simulink model "ards_model"  (R2020b)
settings: Solver=VariableStepAuto  StartTime=0.0  StopTime=480  MaxStep=0.2  RelTol=1e-3
model workspace: external: MAT-File model_workspace.mat (data not in the file)
values from neighbouring files (symbols this model uses):
  C_a_CO2_0 = 0.54    [model_workspace.mat]
  C_a_O2_0 = 0.1974    [model_workspace.mat]
  C_v_CO2_0 = 0.72    [model_workspace.mat]
  C_v_O2_0 = 0.13    [model_workspace.mat]
  moving_average_period = 5    [model_workspace.mat]
  P_ap_0 = 15    [model_workspace.mat]
  P_as_0 = 105.55    [model_workspace.mat]
  P_default = [105.55 4 15 6]    [model_workspace.mat]
  P_vs_0 = 4    [model_workspace.mat]
  Q_0 = 4.8    [model_workspace.mat]
undefined symbols (not defined in the file or in its folder): cRS, Pinsp, VT
libraries: pid_lib x1
(part 3 of 3)

== system ards_model/main-model/Lung volume model/Inspiratory lung volume derivative (fourier approximation)/Half-wave rectifier ==
  (d)VA : Inport
  2pift : Inport  Port=2
  Add : Sum  Inputs=+-+
  Add2 : Sum  Inputs=+++
  Constant : Constant  Value=1/pi
  Constant1 : Constant  Value=2
  Constant2 : Constant  Value=4
  Constant3 : Constant  Value=6
  Gain : Gain  Gain=1/2
  Gain1 : Gain  Gain=2/pi
  Product1 : Product
  Trigonometric Function : Trigonometry
  summand (k=2) : Subsystem
  summand (k=4) : Subsystem
  summand (k=6) : Subsystem
  out : Outport
  wires:
  Trigonometric Function/1 -> Gain/1
  Gain/1 -> Add/3
  (d)VA/1 -> Product1/2  "A"
  2pift/1 -> summand (k=6)/1(In1), summand (k=4)/1(In1), summand (k=2)/1(In1), Trigonometric Function/1  "omega*t"
  Constant/1 -> Add/1
  Add/1 -> Product1/1
  Product1/1 -> out/1
  Gain1/1 -> Add/2
  Add2/1 -> Gain1/1
  Constant1/1 -> summand (k=2)/2(In2)
  summand (k=2)/1(Out1) -> Add2/1
  summand (k=4)/1(Out1) -> Add2/2
  summand (k=6)/1(Out1) -> Add2/3
  Constant3/1 -> summand (k=6)/2(In2)
  Constant2/1 -> summand (k=4)/2(In2)

== system ards_model/main-model/Predicted Body Weight/IfThenElse/Subsystem1 ==
  in : Inport
  Enable : EnablePort
  out : Outport
  wires:
  in/1 -> out/1

== system ards_model/main-model/Predicted Body Weight/IfThenElse/Subsystem2 ==
  in : Inport
  Enable : EnablePort
  out : Outport
  wires:
  in/1 -> out/1

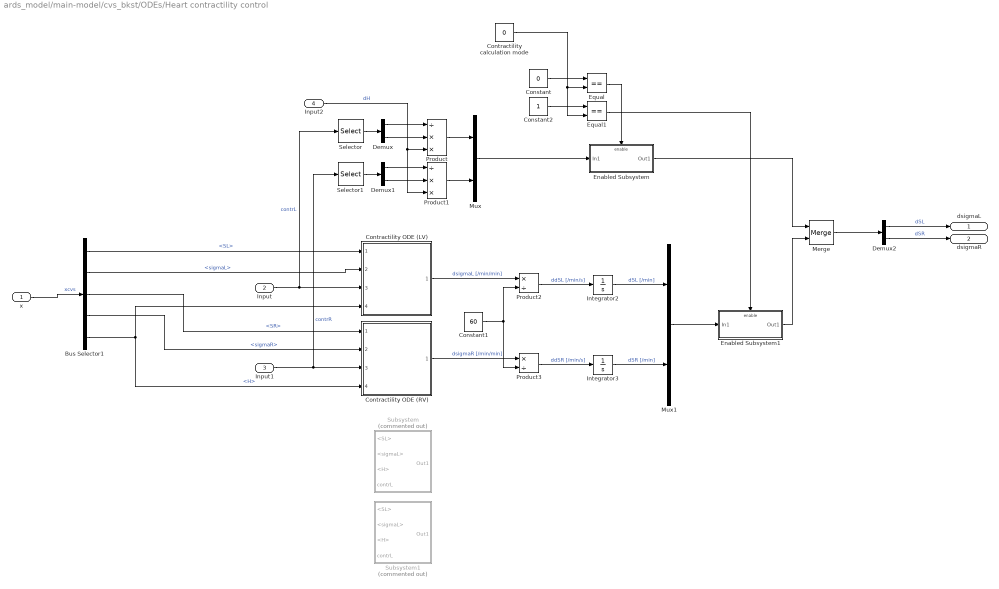
== system ards_model/main-model/cvs_bkst/ODEs/Heart contractility control ==
  x : Inport  OutDataTypeStr=Bus: CardioVascularState
  Input : Inport  Port=2  OutDataTypeStr=double  PortDimensions=3
  Input1 : Inport  Port=3  OutDataTypeStr=double  PortDimensions=3
  Input2 : Inport  Port=4  Unit=1/min^2
  Bus Selector1 : BusSelector  OutputSignals=SL,sigmaL,SR,sigmaR,H
  Constant : Constant  Value=0
  Constant1 : Constant  Value=60
  Constant2 : Constant
  Contractility ODE (LV) : Subsystem  ReferencedSubsystem=cvrs_contractility_control
  Contractility ODE (RV) : Subsystem  ReferencedSubsystem=cvrs_contractility_control
  Contractility calculation mode : Constant  Value=0
  Demux : Demux  Outputs=2
  Demux1 : Demux  Outputs=2
  Demux2 : Demux  Outputs=2
  Enabled Subsystem : Subsystem  TreatAsAtomicUnit=on
  Enabled Subsystem1 : Subsystem  TreatAsAtomicUnit=on
  Equal : RelationalOperator  Operator===  OutDataTypeStr=boolean  RndMeth=Simplest
  Equal1 : RelationalOperator  Operator===  OutDataTypeStr=boolean  RndMeth=Simplest
  Integrator2 : Integrator
  Integrator3 : Integrator
  Merge : Merge
  Mux : Mux  Inputs=2
  Mux1 : Mux  Inputs=2
  Product : Product  Inputs=/**
  Product1 : Product  Inputs=/**
  Product2 : Product  Inputs=*/
  Product3 : Product  Inputs=*/
  Selector : Selector  InputPortWidth=3  IndexOptions=Index vector (dialog)  Indices=[1 2]  OutputSizes=1
  Selector1 : Selector  InputPortWidth=3  IndexOptions=Index vector (dialog)  Indices=[1 2]  OutputSizes=1
  Subsystem : Subsystem  Commented=on
  Subsystem1 : Subsystem  Commented=on
  dsigmaL : Outport  Unit=mmHg/min
  dsigmaR : Outport  Port=2  Unit=mmHg/min
  wires:
  Integrator3/1 -> Mux1/2  "dSR [/min]"
  Integrator2/1 -> Mux1/1  "dSL [/min]"
  Product3/1 -> Integrator3/1  "ddSR [/min/s]"
  Product2/1 -> Integrator2/1  "ddSL [/min/s]"
  Constant1/1 -> Product2/2, Product3/2
  Bus Selector1/3 -> Contractility ODE (RV)/1  "<SR>"
  Input1/1 -> Selector1/1, Contractility ODE (RV)/3  "contrR"
  Contractility ODE (LV)/1 -> Product2/1  "dsigmaL [/min/min]"
  Input/1 -> Selector/1, Contractility ODE (LV)/3  "contrL"
  Bus Selector1/1 -> Contractility ODE (LV)/1  "<SL>"
  Contractility ODE (RV)/1 -> Product3/1  "dsigmaR [/min/min]"
  x/1 -> Bus Selector1/1  "xcvs"
  Bus Selector1/4 -> Contractility ODE (RV)/2  "<sigmaR>"
  Bus Selector1/2 -> Contractility ODE (LV)/2  "<sigmaL>"
  Bus Selector1/5 -> Contractility ODE (LV)/4, Contractility ODE (RV)/4  "<H>"
  Selector/1 -> Demux/1
  Demux/1 -> Product/1
  Demux/2 -> Product/2
  Demux1/2 -> Product1/2
  Demux1/1 -> Product1/1
  Selector1/1 -> Demux1/1
  Product/1 -> Mux/1
  Product1/1 -> Mux/2
  Mux/1 -> Enabled Subsystem/1(In1)
  Mux1/1 -> Enabled Subsystem1/1(In1)
  Equal/1 -> Enabled Subsystem/Enable
  Equal1/1 -> Enabled Subsystem1/Enable
  Enabled Subsystem/1(Out1) -> Merge/1
  Enabled Subsystem1/1(Out1) -> Merge/2
  Demux2/1 -> dsigmaL/1  "dSL"
  Demux2/2 -> dsigmaR/1  "dSR"
  Merge/1 -> Demux2/1
  Constant/1 -> Equal/1
  Constant2/1 -> Equal1/1
  Contractility calculation mode/1 -> Equal1/2, Equal/2
  Input2/1 -> Product1/3, Product/3  "dH"

== system ards_model/main-model/cvs_bkst/ODEs/Heart rate control ==
  <Pas> : Inport  Unit=mmHg
  ABP error term : Subsystem
  Lung-to-carotid delay [BKST] ch. 2.3.1 : TransportDelay  DelayTime=6
  PID Controller : pid_lib/PID Controller  Controller=PID  Form=Parallel  TimeDomain=Continuous-time  UseExternalTs=off  SampleTime=-1  IntegratorMethod=Forward Euler  FilterMethod=Forward Euler  ControllerParametersSource=internal  P=0.5  I=0  D=-0.3  UseFilter=on  N=100  TunerSelectOption=Transfer Function Based (PID Tuner App)  InitialConditionSource=internal  InitialConditionForIntegrator=0  InitialConditionForFilter=0  DifferentiatorICPrevScaledInput=0  ExternalReset=none  TrackingMode=off  Kt=1  LimitOutput=off  SatLimitsSource=internal  UpperSaturationLimit=inf  LowerSaturationLimit=-inf  LinearizeAsGain=on  AntiWindupMode=none  Kb=1  POutMin=[]  POutMax=[]  IOutMin=[]  IOutMax=[]  DOutMin=[]  DOutMax=[]  NOutMin=[]  NOutMax=[]  SumOutMin=[]  SumOutMax=[]  SaturationOutMin=[]  SaturationOutMax=[]  PParamMin=[]  PParamMax=[]  IParamMin=[]  IParamMax=[]  DParamMin=[]  DParamMax=[]  NParamMin=[]  NParamMax=[]  KbParamMin=[]  KbParamMax=[]  KtParamMin=[]  KtParamMax=[]  KbOutMin=[]  KbOutMax=[]  KtOutMin=[]  KtOutMax=[]  IntegratorOutMin=[]  IntegratorOutMax=[]  FilterOutMin=[]  FilterOutMax=[]  SumI1OutMin=[]  SumI1OutMax=[]  SumI2OutMin=[]  SumI2OutMax=[]  SumI3OutMin=[]  SumI3OutMax=[]  SumI4OutMin=[]  SumI4OutMax=[]  SumDOutMin=[]  SumDOutMax=[]  DifferentiatorOutMin=[]  DifferentiatorOutMax=[]  FilterDiffOutCoefMin=[]  FilterDiffOutCoefMax=[]  ReciprocalOutMin=[]  ReciprocalOutMax=[]  SumDenOutMin=[]  SumDenOutMax=[]  SumNumOutMin=[]  SumNumOutMax=[]  DivideOutMin=[]  DivideOutMax=[]  UdiffTsProdOutMin=[]  UdiffTsProdOutMax=[]  NTsProdOutMin=[]  NTsProdOutMax=[]  UintegralTsProdOutMin=[]  UintegralTsProdOutMax=[]  UngainTsProdOutMin=[]  UngainTsProdOutMax=[]  IntegratorContinuousStateAttributes=''  IntegratorStateMustResolveToSignalObject=off  IntegratorRTWStateStorageClass=Auto  FilterContinuousStateAttributes=''  FilterStateMustResolveToSignalObject=off  FilterRTWStateStorageClass=Auto  ParallelPVariant=InternalParameters  IdealPVariant=Disabled  IVariant=InternalParameters  DVariant=InternalParameters  IntegratorVariant=Continuous  SatVariant=Disabled  AWVariant=Passthrough  PCopyVariant=Disabled  TRVariant=Disabled  FdbkBlocksVariant=Forward  IdealPFdbkVariant=Disabled  SatFdbkVariant=Disabled  DerivativeFilterVariant=ContFilter  NVariant=InternalParameters  NCopyVariant=Disabled  FilterICVariant=InternalICsFilter  IntegratorICVariant=InternalICs  ExternalResetVariant=Disabled  TRSumVariant=Passthrough  SumFdbkVariant=Disabled  SumVariant=Sum_PID  TsampFilterVariant=InternalTs  TsampNgainVariant=Passthrough  TsampIntegralVariant=Passthrough  ExternalSaturationOutDataTypeStr=Inherit: Same as second input
  Pas : Constant  Value=105.5
  dH [/min] : Outport  Unit=1/min^2
  wires:
  ABP error term/1(Out1) -> Lung-to-carotid delay [BKST] ch. 2.3.1/1
  PID Controller/1 -> dH [/min]/1  "dH [/min]"
  <Pas>/1 -> ABP error term/1(<Pas>)  "Pas"
  Pas/1 -> ABP error term/2(<Pas>1)
  Lung-to-carotid delay [BKST] ch. 2.3.1/1 -> PID Controller/1

== system ards_model/main-model/cvs_bkst/ODEs/Systemic vascular resistance control ==
  xcvsExt : Inport  OutDataTypeStr=Bus: CardioVascularStateExtended
  Ca;O2 : Inport  Port=2  Unit=1
  Ca;O1 : Inport  Port=3  Unit=1
  -MR_;O2 : Inport  Port=4  Unit=L/min
  Apesk [mmHg*min/L] : Constant  Value=178
  Bus Selector : BusSelector  OutputSignals=Qs,Pas,Pvs
  Constant3 : Constant  Value=0
  Derivative : Derivative
  Divide1 : Product  Inputs=*/
  K [L] : Constant  Value=15.9591
  Product : Product
  Product1 : Product
  Product2 : Product
  Subsystem : Subsystem
  Subtract : Sum  Inputs=+-
  Subtract1 : Sum  Inputs=+-
  Subtract2 : Sum  Inputs=+-
  Rs1 : Outport  Unit=mmHg/L
  wires:
  -MR_;O2/1 -> Subtract1/2  "-MR_;O2"
  Product1/1 -> Subtract2/1
  Product/1 -> Subtract1/1
  Subtract2/1 -> Divide1/1
  Subtract1/1 -> Product1/2
  Subtract/1 -> Subtract2/2  "deltaP"
  Ca;O2/1 -> Product/1  "Ca;O2"
  Bus Selector/2 -> Subtract/1  "<Pas>"
  Bus Selector/1 -> Product/2  "<Qs>"
  Apesk [mmHg*min/L]/1 -> Product1/1, Product2/1  "Apesk"
  K [L]/1 -> Divide1/2  "K"
  xcvsExt/1 -> Bus Selector/1  "xcvsExt"
  Bus Selector/3 -> Subtract/2  "<Pvs>"
  Ca;O1/1 -> Derivative/1  "Cv;O2"
  Derivative/1 -> Product2/2
  Constant3/1 -> Subsystem/1(dRs [0])
  Product2/1 -> Subsystem/2(dRs [v])  "dRs [v]"
  Divide1/1 -> Subsystem/3(dRs [a])  "dRs [a]"
  Subsystem/1(dRs) -> Rs1/1  "dRs"

== system ards_model/main-model/cvs_bkst/ODEs/Vessel pressure control (ap) ==
  Qin : Inport
  Qout : Inport  Port=2
  c_ : Inport  Port=3
  Add4 : Sum  Inputs=+-
  Product4 : Product  Inputs=*/
  dP_ : Outport
  wires:
  Qout/1 -> Add4/2
  Product4/1 -> dP_/1  "dP_"
  c_/1 -> Product4/2
  Qin/1 -> Add4/1
  Add4/1 -> Product4/1

== system ards_model/main-model/cvs_bkst/ODEs/Vessel pressure control (as) ==
  Qin : Inport
  Qout : Inport  Port=2
  c_ : Inport  Port=3
  Add4 : Sum  Inputs=+-
  Product4 : Product  Inputs=*/
  dP_ : Outport
  wires:
  Add4/1 -> Product4/1
  Qin/1 -> Add4/1
  c_/1 -> Product4/2
  Product4/1 -> dP_/1  "dP_"
  Qout/1 -> Add4/2

== system ards_model/main-model/cvs_bkst/ODEs/Vessel pressure control (vs) ==
  Qin : Inport
  Qout : Inport  Port=2
  c_ : Inport  Port=3
  Add4 : Sum  Inputs=+-
  Product4 : Product  Inputs=*/
  dP_ : Outport
  wires:
  Add4/1 -> Product4/1
  Qin/1 -> Add4/1
  c_/1 -> Product4/2
  Product4/1 -> dP_/1  "dP_"
  Qout/1 -> Add4/2

== system ards_model/main-model/rs_tehrani/ODEs/Ambient air pressure (-H2O) ==
  QT12 : Inport
  PA;H2O [mmHg] : Constant  Value=47
  Subtract : Sum  Inputs=+-
  Output : Outport
  wires:
  QT12/1 -> Subtract/1  "Pamb"
  PA;H2O [mmHg]/1 -> Subtract/2
  Subtract/1 -> Output/1  "Pamb*"

== system ards_model/main-model/rs_tehrani/ODEs/Insipired gas pressures ==
  Pamb* : Inport  Unit=mmHg
  Fi;O2 : Inport  Port=2  Unit=1
  Fi;CO2 : Inport  Port=3  Unit=1
  Product : Product  Inputs=**
  Product1 : Product  Inputs=**
  Pi;O2 : Outport  Unit=mmHg
  Pi;CO2 : Outport  Port=2  Unit=mmHg
  wires:
  Fi;CO2/1 -> Product1/2
  Fi;O2/1 -> Product/2
  Product/1 -> Pi;O2/1  "Pi;O2"
  Product1/1 -> Pi;CO2/1  "Pi;CO2"
  Pamb*/1 -> Product/1, Product1/1

== system ards_model/main-model/rs_tehrani/ODEs/lung_compartment ==
  Pamb* : Inport  Unit=mmHg
  dv1 : Inport  Port=2  Unit=L
  dv : Inport  Port=3  Unit=L/s
  Pi;O2 : Inport  Port=4  Unit=mmHg
  Pi;CO2 : Inport  Port=5  Unit=mmHg
  Input : Inport  Port=6  OutDataTypeStr=Bus: RespiratoryStateExtended
  dv4 : Inport  Port=7  OutDataTypeStr=Bus: BloodGasFlow
  Bus Selector : BusSelector  OutputSignals=CaxO2,PaxO2
  Bus Selector1 : BusSelector  OutputSignals=CaxCO2,PaxCO2
  Bus Selector2 : BusSelector  OutputSignals=Q,C_O2
  Bus Selector3 : BusSelector  OutputSignals=Q,C_CO2
  CO2 : Subsystem  ReferencedSubsystem=tehrani_alv_mass_balance_v5
  Input1 : InportShadow  Port=6  OutDataTypeStr=Bus: RespiratoryStateExtended
  O2 : Subsystem  ReferencedSubsystem=tehrani_alv_mass_balance_v5
  PA-a;CO2 : Constant  Value=0
  PA-a;O2 : Constant  Value=4
  dv2 : InportShadow  Port=7  OutDataTypeStr=Bus: BloodGasFlow
  Output : Outport  Unit=mmHg/s
  Output1 : Outport  Port=2  Unit=mmHg/s
  wires:
  Bus Selector2/1 -> O2/1  "<Q>"
  Bus Selector2/2 -> O2/2  "<C_O2>"
  Pi;CO2/1 -> CO2/6  "Pi;CO2"
  Bus Selector1/1 -> CO2/3  "<CaxCO2>"
  dv4/1 -> Bus Selector2/1  "inpp*"
  Input1/1 -> Bus Selector1/1  "xrsExt"
  dv2/1 -> Bus Selector3/1  "inpp*"
  Bus Selector3/1 -> CO2/1  "<Q>"
  Bus Selector3/2 -> CO2/2  "<C_CO2>"
  Input/1 -> Bus Selector/1  "xrsExt"
  Bus Selector1/2 -> CO2/4  "<PaxCO2>"
  O2/1 -> Output/1  "dPax;O2"
  Bus Selector/1 -> O2/3  "<CaxO2>"
  PA-a;CO2/1 -> CO2/9  "PA-a;CO2"
  CO2/1 -> Output1/1  "dPax;CO2"
  Bus Selector/2 -> O2/4  "<PaxO2>"
  dv1/1 -> CO2/7, O2/7  "v"
  Pi;O2/1 -> O2/6  "Pi;O2"
  dv/1 -> CO2/8, O2/8  "dv+"
  Pamb*/1 -> CO2/5, O2/5  "Pamb*"
  PA-a;O2/1 -> O2/9  "PA-a;O2"

== system ards_model/ards_classification/Berlin definition/ards_level/ards_level_string/Subsystem ==
  in : Inport
  Enable : EnablePort
  out : Outport
  wires:
  in/1 -> out/1

== system ards_model/ards_classification/Berlin definition/ards_level/ards_level_string/Subsystem1 ==
  in : Inport
  Enable : EnablePort
  out : Outport
  wires:
  in/1 -> out/1

== system ards_model/ards_classification/Berlin definition/ards_level/ards_level_string/Subsystem2 ==
  in : Inport
  Enable : EnablePort
  out : Outport
  wires:
  in/1 -> out/1

== system ards_model/ards_classification/Berlin definition/ards_level/ards_level_string/Subsystem3 ==
  in : Inport
  Enable : EnablePort
  out : Outport
  wires:
  in/1 -> out/1

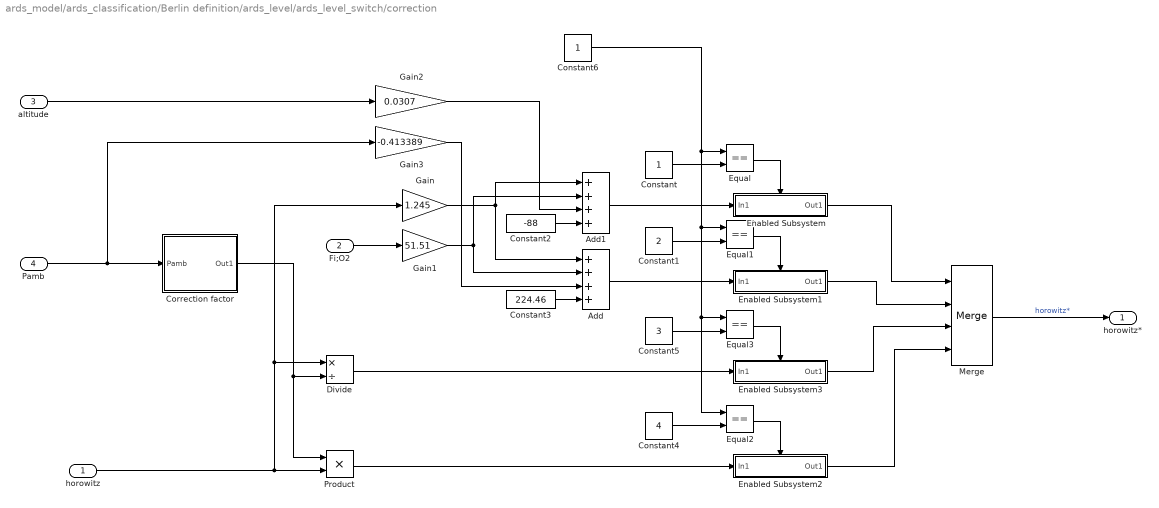
== system ards_model/ards_classification/Berlin definition/ards_level/ards_level_switch/correction ==
  horowitz : Inport
  Fi;O2 : Inport  Port=2
  altitude : Inport  Port=3
  Pamb : Inport  Port=4
  Add : Sum  Inputs=++++
  Add1 : Sum  Inputs=++++
  Constant : Constant
  Constant1 : Constant  Value=2
  Constant2 : Constant  Value=-88
  Constant3 : Constant  Value=224.46
  Constant4 : Constant  Value=4
  Constant5 : Constant  Value=3
  Constant6 : Constant
  Correction factor : Subsystem
  Divide : Product  Inputs=*/
  Enabled Subsystem : Subsystem  TreatAsAtomicUnit=on
  Enabled Subsystem1 : Subsystem  TreatAsAtomicUnit=on
  Enabled Subsystem2 : Subsystem  TreatAsAtomicUnit=on
  Enabled Subsystem3 : Subsystem  TreatAsAtomicUnit=on
  Equal{,1..3} (4 alike) : RelationalOperator  Operator===  OutDataTypeStr=boolean  RndMeth=Simplest
  Gain : Gain  Gain=1.245
  Gain1 : Gain  Gain=51.51
  Gain2 : Gain  Gain=0.0307
  Gain3 : Gain  Gain=-0.413389
  Merge : Merge  Inputs=4
  Product : Product
  horowitz* : Outport
  wires:
  Correction factor/1(Out1) -> Divide/2, Product/1
  Constant1/1 -> Equal1/2
  Constant/1 -> Equal/2
  Constant6/1 -> Equal2/1, Equal3/1, Equal1/1, Equal/1
  Gain1/1 -> Add1/2, Add/2
  horowitz/1 -> Gain/1, Divide/1, Product/2
  Enabled Subsystem/1(Out1) -> Merge/1
  Gain3/1 -> Add/3
  Constant4/1 -> Equal2/2
  Pamb/1 -> Gain3/1, Correction factor/1(Pamb)
  Enabled Subsystem2/1(Out1) -> Merge/4
  Constant2/1 -> Add1/4
  Merge/1 -> horowitz*/1  "horowitz*"
  altitude/1 -> Gain2/1
  Gain/1 -> Add/1, Add1/1
  Add/1 -> Enabled Subsystem1/1(In1)
  Divide/1 -> Enabled Subsystem3/1(In1)
  Enabled Subsystem3/1(Out1) -> Merge/3
  Constant3/1 -> Add/4
  Equal1/1 -> Enabled Subsystem1/Enable
  Add1/1 -> Enabled Subsystem/1(In1)
  Gain2/1 -> Add1/3
  Product/1 -> Enabled Subsystem2/1(In1)
  Equal2/1 -> Enabled Subsystem2/Enable
  Equal3/1 -> Enabled Subsystem3/Enable
  Equal/1 -> Enabled Subsystem/Enable
  Constant5/1 -> Equal3/2
  Enabled Subsystem1/1(Out1) -> Merge/2
  Fi;O2/1 -> Gain1/1

== system ards_model/main-model/Lung volume model/Inspiratory lung volume derivative (fourier approximation)/Half-wave rectifier/summand (k=2) ==
  In1 : Inport
  In2 : Inport  Port=2
  Add1 : Sum  Inputs=+-
  Constant2 : Constant
  Product : Product
  Product3 : Product  Inputs=*/
  Square : Math  Operator=square  SaturateOnIntegerOverflow=on
  Trigonometric Function1 : Trigonometry  Operator=cos
  Out1 : Outport
  wires:
  Add1/1 -> Product3/2
  Trigonometric Function1/1 -> Product3/1
  Square/1 -> Add1/1
  In1/1 -> Product/1  "omega*t"
  In2/1 -> Product/2, Square/1  "n"
  Product/1 -> Trigonometric Function1/1
  Product3/1 -> Out1/1
  Constant2/1 -> Add1/2

== system ards_model/main-model/Lung volume model/Inspiratory lung volume derivative (fourier approximation)/Half-wave rectifier/summand (k=4) ==
  In1 : Inport
  In2 : Inport  Port=2
  Add1 : Sum  Inputs=+-
  Constant2 : Constant
  Product : Product
  Product3 : Product  Inputs=*/
  Square : Math  Operator=square  SaturateOnIntegerOverflow=on
  Trigonometric Function1 : Trigonometry  Operator=cos
  Out1 : Outport
  wires:
  Constant2/1 -> Add1/2
  Product3/1 -> Out1/1
  Product/1 -> Trigonometric Function1/1
  In2/1 -> Square/1, Product/2  "n"
  In1/1 -> Product/1  "omega*t"
  Square/1 -> Add1/1
  Trigonometric Function1/1 -> Product3/1
  Add1/1 -> Product3/2

== system ards_model/main-model/Lung volume model/Inspiratory lung volume derivative (fourier approximation)/Half-wave rectifier/summand (k=6) ==
  In1 : Inport
  In2 : Inport  Port=2
  Add1 : Sum  Inputs=+-
  Constant2 : Constant
  Product : Product
  Product3 : Product  Inputs=*/
  Square : Math  Operator=square  SaturateOnIntegerOverflow=on
  Trigonometric Function1 : Trigonometry  Operator=cos
  Out1 : Outport
  wires:
  Add1/1 -> Product3/2
  Trigonometric Function1/1 -> Product3/1
  Square/1 -> Add1/1
  In1/1 -> Product/1  "omega*t"
  In2/1 -> Product/2, Square/1  "n"
  Product/1 -> Trigonometric Function1/1
  Product3/1 -> Out1/1
  Constant2/1 -> Add1/2

== system ards_model/main-model/cvs_bkst/ODEs/Heart contractility control/Enabled Subsystem ==
  In1 : Inport
  Enable : EnablePort
  Out1 : Outport
  wires:
  In1/1 -> Out1/1

== system ards_model/main-model/cvs_bkst/ODEs/Heart contractility control/Enabled Subsystem1 ==
  In1 : Inport
  Enable : EnablePort
  Out1 : Outport
  wires:
  In1/1 -> Out1/1

== system ards_model/main-model/cvs_bkst/ODEs/Heart contractility control/Subsystem ==
  <SL> : Inport
  <sigmaL> : Inport  Port=2
  <H> : Inport  Port=3
  contrL : Inport  Port=4
  Add : Sum  Inputs=-+-
  Demux : Demux  Outputs=3
  Derivative : Derivative
  Divide : Product  Inputs=*/
  Gain : Gain  Commented=through  Gain=60
  Product : Product
  Product1 : Product
  Out1 : Outport
  wires:
  contrL/1 -> Demux/1
  Gain/1 -> Add/3
  Product1/1 -> Add/2
  Product/1 -> Add/1
  Add/1 -> Divide/1
  Demux/1 -> Product/1
  <SL>/1 -> Product/2
  Demux/2 -> Product1/1
  Demux/3 -> Divide/2
  Derivative/1 -> Gain/1
  <sigmaL>/1 -> Derivative/1
  Divide/1 -> Out1/1
  <H>/1 -> Product1/2

== system ards_model/main-model/cvs_bkst/ODEs/Heart contractility control/Subsystem1 ==
  <SL> : Inport
  <sigmaL> : Inport  Port=2
  <H> : Inport  Port=3
  contrL : Inport  Port=4
  Add : Sum  Inputs=-+-
  Demux : Demux  Outputs=3
  Derivative : Derivative
  Divide : Product  Inputs=*/
  Gain : Gain  Commented=through  Gain=60
  Product : Product
  Product1 : Product
  Out1 : Outport
  wires:
  <H>/1 -> Product1/2
  Divide/1 -> Out1/1
  <sigmaL>/1 -> Derivative/1
  Derivative/1 -> Gain/1
  Demux/3 -> Divide/2
  Demux/2 -> Product1/1
  <SL>/1 -> Product/2
  Demux/1 -> Product/1
  Add/1 -> Divide/1
  Product/1 -> Add/1
  Product1/1 -> Add/2
  Gain/1 -> Add/3
  contrL/1 -> Demux/1

== system ards_model/main-model/cvs_bkst/ODEs/Heart rate control/ABP error term ==
  <Pas> : Inport  Unit=mmHg
  <Pas>1 : Inport  Port=2  Unit=mmHg
  Subtract : Sum  Inputs=-+
  Out1 : Outport
  wires:
  <Pas>/1 -> Subtract/1  "Pas"
  <Pas>1/1 -> Subtract/2  "Pas^"
  Subtract/1 -> Out1/1  "s"

== system ards_model/main-model/cvs_bkst/ODEs/Systemic vascular resistance control/Subsystem ==
  dRs [0] : Inport
  dRs [v] : Inport  Port=2
  dRs [a] : Inport  Port=3
  Constant : Constant  Value=0
  Constant1 : Constant
  Constant2 : Constant  Value=2
  Equal : RelationalOperator  Operator===  OutDataTypeStr=boolean  RndMeth=Simplest
  Equal1 : RelationalOperator  Operator===  OutDataTypeStr=boolean  RndMeth=Simplest
  Equal2 : RelationalOperator  Operator===  OutDataTypeStr=boolean  RndMeth=Simplest
  Merge : Merge  Inputs=3
  Rs calculation mode : Constant  Value=2
  Subsystem1 : Subsystem
  Subsystem2 : Subsystem
  Subsystem3 : Subsystem
  dRs : Outport  Unit=mmHg/L
  wires:
  Subsystem3/1(out) -> Merge/1
  Constant2/1 -> Equal2/1
  Constant1/1 -> Equal1/1
  dRs [a]/1 -> Subsystem1/1(in)  "dRs;mode2"
  Equal1/1 -> Subsystem2/Enable
  Subsystem2/1(out) -> Merge/2
  Constant/1 -> Equal/1
  Equal/1 -> Subsystem3/Enable
  dRs [0]/1 -> Subsystem3/1(in)  "dRs;mode0"
  Rs calculation mode/1 -> Equal2/2, Equal1/2, Equal/2
  Merge/1 -> dRs/1  "dRs"
  Equal2/1 -> Subsystem1/Enable
  Subsystem1/1(out) -> Merge/3
  dRs [v]/1 -> Subsystem2/1(in)  "dRs;mode1"

== system ards_model/ards_classification/Berlin definition/ards_level/ards_level_switch/correction/Correction factor ==
  Pamb : Inport  Unit=mmHg
  Constant : Constant  Value=760
  Divide2 : Product  Inputs=*/
  Out1 : Outport  Unit=1
  wires:
  Constant/1 -> Divide2/1
  Divide2/1 -> Out1/1  "a"
  Pamb/1 -> Divide2/2  "Pamb"

== system ards_model/ards_classification/Berlin definition/ards_level/ards_level_switch/correction/Enabled Subsystem ==
  In1 : Inport
  Enable : EnablePort
  Out1 : Outport
  wires:
  In1/1 -> Out1/1

== system ards_model/ards_classification/Berlin definition/ards_level/ards_level_switch/correction/Enabled Subsystem1 ==
  In1 : Inport
  Enable : EnablePort
  Out1 : Outport
  wires:
  In1/1 -> Out1/1

== system ards_model/ards_classification/Berlin definition/ards_level/ards_level_switch/correction/Enabled Subsystem2 ==
  In1 : Inport
  Enable : EnablePort
  Out1 : Outport
  wires:
  In1/1 -> Out1/1

== system ards_model/ards_classification/Berlin definition/ards_level/ards_level_switch/correction/Enabled Subsystem3 ==
  In1 : Inport
  Enable : EnablePort
  Out1 : Outport
  wires:
  In1/1 -> Out1/1

== system ards_model/main-model/cvs_bkst/ODEs/Systemic vascular resistance control/Subsystem/Subsystem1 ==
  in : Inport
  Enable : EnablePort
  out : Outport
  wires:
  in/1 -> out/1

== system ards_model/main-model/cvs_bkst/ODEs/Systemic vascular resistance control/Subsystem/Subsystem2 ==
  in : Inport
  Enable : EnablePort
  out : Outport
  wires:
  in/1 -> out/1

== system ards_model/main-model/cvs_bkst/ODEs/Systemic vascular resistance control/Subsystem/Subsystem3 ==
  in : Inport
  Enable : EnablePort
  out : Outport
  wires:
  in/1 -> out/1
